simulink model "yourcontroller"  (R2023a)
settings: Solver=VariableStepAuto  StartTime=0.0  StopTime=10.0  RelTol=1e-3
libraries: simulink_extras x4
settings Model: Creator=james  LastModifiedBy=james

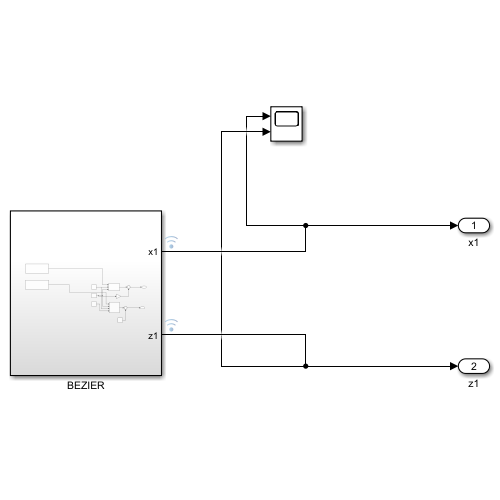
[thumbnail: Simulink's stored preview of the top-level diagram]
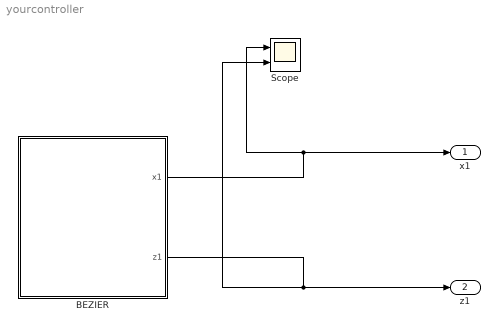
== system yourcontroller ==
  BEZIER : Subsystem
  Scope : Scope  NumInputPorts=2
  x1 : Outport  VectorParamsAs1DForOutWhenUnconnected=off
  z1 : Outport  Port=2  VectorParamsAs1DForOutWhenUnconnected=off
  wires:
  BEZIER/1(x1) -> x1/1, Scope/1
  BEZIER/2(z1) -> z1/1, Scope/2

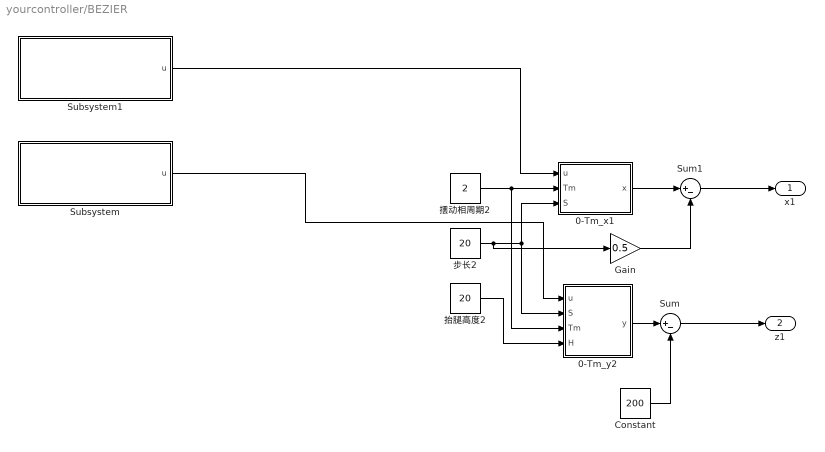
== system yourcontroller/BEZIER ==
  0-Tm_x1 : MATLAB Function  TreatAsAtomicUnit=on
  0-Tm_y2 : MATLAB Function  TreatAsAtomicUnit=on
  Constant : Constant  Value=200
  Gain : Gain  Gain=0.5
  Subsystem : Subsystem
  Subsystem1 : Subsystem
  Sum : Sum  Inputs=|+-
  Sum1 : Sum  Inputs=|+-
  抬腿高度2 : Constant  Value=20
  摆动相周期2 : Constant  Value=2
  步长2 : Constant  Value=20
  x1 : Outport  VectorParamsAs1DForOutWhenUnconnected=off
  z1 : Outport  Port=2  VectorParamsAs1DForOutWhenUnconnected=off
  wires:
  0-Tm_x1/1(x) -> Sum1/1
  抬腿高度2/1 -> 0-Tm_y2/4(H)
  步长2/1 -> Gain/1, 0-Tm_y2/2(S), 0-Tm_x1/3(S)
  Subsystem/1(u) -> 0-Tm_y2/1(u)
  摆动相周期2/1 -> 0-Tm_y2/3(Tm), 0-Tm_x1/2(Tm)
  Subsystem1/1(u) -> 0-Tm_x1/1(u)
  0-Tm_y2/1(y) -> Sum/1
  Sum/1 -> z1/1
  Constant/1 -> Sum/2
  Gain/1 -> Sum1/2
  Sum1/1 -> x1/1

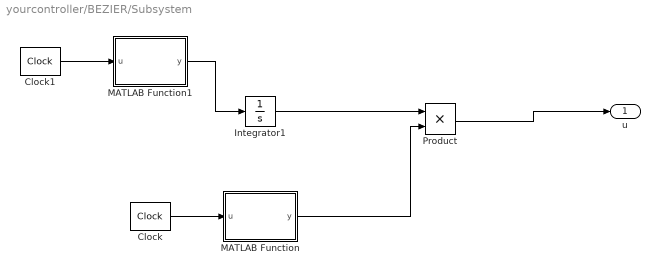
== system yourcontroller/BEZIER/Subsystem ==
  Clock : simulink_extras/Flip Flops/Clock  period=4
  Clock1 : simulink_extras/Flip Flops/Clock  period=2
  Integrator1 : Integrator
  MATLAB Function : MATLAB Function  TreatAsAtomicUnit=on
  MATLAB Function1 : MATLAB Function  TreatAsAtomicUnit=on
  Product : Product
  u : Outport  VectorParamsAs1DForOutWhenUnconnected=off
  wires:
  MATLAB Function1/1(y) -> Integrator1/1
  Clock1/1 -> MATLAB Function1/1(u)
  MATLAB Function/1(y) -> Product/2
  Clock/1 -> MATLAB Function/1(u)
  Integrator1/1 -> Product/1
  Product/1 -> u/1

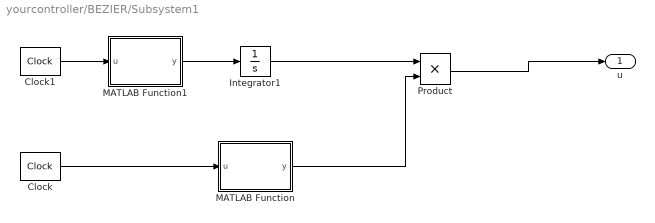
== system yourcontroller/BEZIER/Subsystem1 ==
  Clock : simulink_extras/Flip Flops/Clock  period=8
  Clock1 : simulink_extras/Flip Flops/Clock  period=4
  Integrator1 : Integrator
  MATLAB Function : MATLAB Function  TreatAsAtomicUnit=on
  MATLAB Function1 : MATLAB Function  TreatAsAtomicUnit=on
  Product : Product
  u : Outport  VectorParamsAs1DForOutWhenUnconnected=off
  wires:
  MATLAB Function1/1(y) -> Integrator1/1
  Clock1/1 -> MATLAB Function1/1(u)
  MATLAB Function/1(y) -> Product/2
  Clock/1 -> MATLAB Function/1(u)
  Integrator1/1 -> Product/1
  Product/1 -> u/1

== matlab function yourcontroller/BEZIER/0-Tm_x1 ==
  data: u input; x output; Tm input; S input
function x = fcn(u,Tm,S)

if u>0
    x =S*(u/Tm-1/(2*pi)*sin(2*pi*u/Tm));
else 
    u=-u;
     x =S*(u/Tm-1/(2*pi)*sin(2*pi*u/Tm));
end

== matlab function yourcontroller/BEZIER/0-Tm_y2 ==
  data: u input; y output; S input; Tm input; H input
function y = fcn(u,S,Tm,H)

n=4;
if u>0
    y=2*H*(u/Tm-1/(n*pi)*sin(n*pi*u/Tm)).*(u>=0&u<Tm/2)+2*H*(1-u/Tm+1/(n*pi)*sin(n*pi*u/Tm)).*(u>=Tm/2&u<Tm);;
else 
    y=0;
end

== matlab function yourcontroller/BEZIER/Subsystem/MATLAB Function ==
  data: u input; y output
function y = fcn(u)
if u==0
    y = -1;
else
    y=1;
end
end

== matlab function yourcontroller/BEZIER/Subsystem/MATLAB Function1 ==
  data: u input; y output
function y = fcn(u)
if u==0
    y = -1;
else
    y=1;
end
end

== matlab function yourcontroller/BEZIER/Subsystem1/MATLAB Function ==
  data: u input; y output
function y = fcn(u)
if u==0
    y = -1;
else
    y=1;
end
end

== matlab function yourcontroller/BEZIER/Subsystem1/MATLAB Function1 ==
  data: u input; y output
function y = fcn(u)
if u==0
    y = -1;
else
    y=1;
end
end
